simulink model "Gerador_de_dados_local"  (R2013a)
settings: Solver=FixedStepDiscrete  StartTime=0.0  StopTime=10.0  RelTol=1e-3
values from neighbouring files (symbols this model uses):
  T = 1    [Variaveis.mat]
undefined symbols (not defined in the file or in its folder): St
settings Model: Creator=Élio  LastModifiedBy=Élio

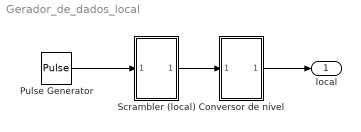
== system Gerador_de_dados_local ==
  Conversor de nível : Subsystem
  Pulse Generator : DiscretePulseGenerator  PulseType=Time based  Period=2*T  PulseWidth=50  SampleTime=St
  Scrambler (local) : Subsystem
  local : Outport
  wires:
  Pulse Generator/1 -> Scrambler (local)/1(In1)
  Scrambler (local)/1(Out1) -> Conversor de nível/1(In2)
  Conversor de nível/1(Out2) -> local/1

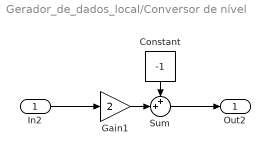
== system Gerador_de_dados_local/Conversor de nível ==
  In2 : Inport
  Constant : Constant  Value=-1
  Gain1 : Gain  Gain=2
  Sum : Sum  Inputs=++|
  Out2 : Outport
  wires:
  In2/1 -> Gain1/1
  Sum/1 -> Out2/1
  Gain1/1 -> Sum/2
  Constant/1 -> Sum/1

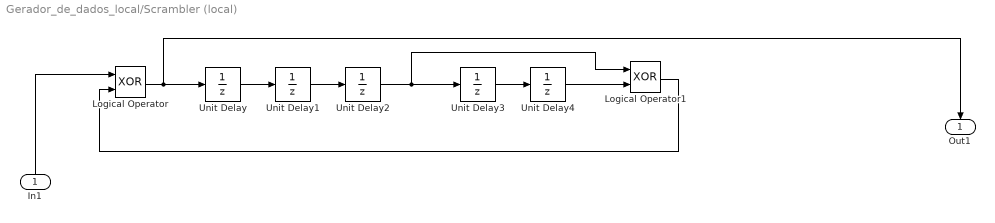
== system Gerador_de_dados_local/Scrambler (local) ==
  In1 : Inport
  Logical Operator : Logic  Operator=XOR  AllPortsSameDT=off  OutDataTypeStr=fixdt(1,16)
  Logical Operator1 : Logic  Operator=XOR  AllPortsSameDT=off  OutDataTypeStr=boolean
  Unit Delay{,1..4} (5 alike) : UnitDelay  SampleTime=-1
  Out1 : Outport
  wires:
  In1/1 -> Logical Operator/1
  Logical Operator/1 -> Out1/1, Unit Delay/1
  Unit Delay/1 -> Unit Delay1/1
  Logical Operator1/1 -> Logical Operator/2
  Unit Delay3/1 -> Unit Delay4/1
  Unit Delay4/1 -> Logical Operator1/2
  Unit Delay1/1 -> Unit Delay2/1
  Unit Delay2/1 -> Logical Operator1/1, Unit Delay3/1
